simulink model "Ornek2_4"  (R2021b)
settings: Solver=VariableStepAuto  StartTime=0.0  StopTime=10  RelTol=1e-3
settings Model: Creator=MONSTER  LastModifiedBy=MONSTER

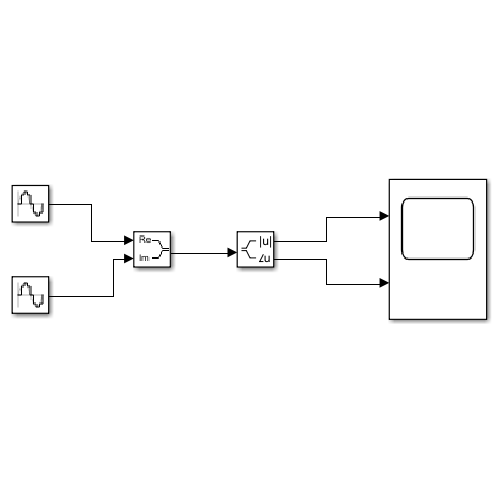
[thumbnail: Simulink's stored preview of the top-level diagram]
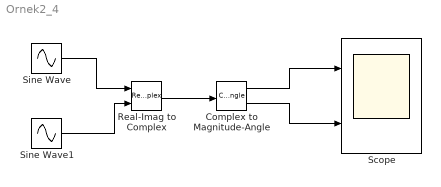
== system Ornek2_4 ==
  Complex to Magnitude-Angle : ComplexToMagnitudeAngle
  Real-Imag to Complex : RealImagToComplex
  Scope : Scope  NumInputPorts=2
  Sine Wave : Sin  Phase=0.5*pi  SampleTime=0.01
  Sine Wave1 : Sin  SampleTime=0.01
  wires:
  Sine Wave/1 -> Real-Imag to Complex/1
  Sine Wave1/1 -> Real-Imag to Complex/2
  Real-Imag to Complex/1 -> Complex to Magnitude-Angle/1
  Complex to Magnitude-Angle/1 -> Scope/1
  Complex to Magnitude-Angle/2 -> Scope/2
